simulink model "untitled"  (R2014b)
settings: Solver=ode45  StartTime=0.0  StopTime=0.01  MaxStep=1e-6  RelTol=1e-3
undefined symbols (not defined in the file or in its folder): powergui
libraries: powerlib x15
settings Model: Creator=JPSOLIV  LastModifiedBy=JPSOLIV

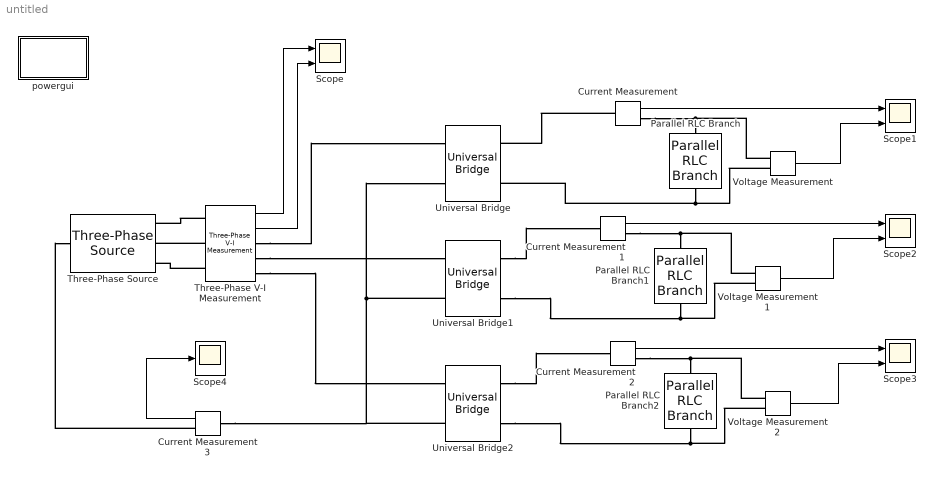
== system untitled ==
  Current Measurement{,1..3} (4 alike) : powerlib/Measurements/Current Measurement  PhasorSimulation=off  OutputType=Complex  PSBequivalent=0
  Parallel RLC Branch : powerlib/Elements/Parallel RLC Branch  LConnTagsString=a  RConnTagsString=__new0  BranchType=RC  Resistance=20  Inductance=1e-3  SetiL0=off  InitialCurrent=0  Capacitance=30e-6  Setx0=off  InitialVoltage=0  Measurements=None
  Parallel RLC Branch1 : powerlib/Elements/Parallel RLC Branch  LConnTagsString=a  RConnTagsString=__new0  BranchType=RC  Resistance=20  Inductance=1e-3  SetiL0=off  InitialCurrent=0  Capacitance=30e-6  Setx0=off  InitialVoltage=0  Measurements=None
  Parallel RLC Branch2 : powerlib/Elements/Parallel RLC Branch  LConnTagsString=a  RConnTagsString=__new0  BranchType=RC  Resistance=20  Inductance=1e-3  SetiL0=off  InitialCurrent=0  Capacitance=30e-6  Setx0=off  InitialVoltage=0  Measurements=None
  Scope{,1..3} (4 alike) : Scope  NumInputPorts=2
      Scope settings: YMin=-600~-200  YMax=400~200
      Scope1 settings: YMin=-0.00169333~0  YMax=20~200
      Scope2 settings: YMin=-5~-5  YMax=5~5  SaveName=ScopeData2
      Scope3 settings: YMin=-5~-5  YMax=5~5  SaveName=ScopeData3
  Scope4 : Scope
      settings: YMin=-10  YMax=15  SaveName=ScopeData4
  Three-Phase V-I Measurement : powerlib/Measurements/Three-Phase V-I Measurement  VoltageMeasurement=phase-to-phase  SetLabelV=off  LabelV=Vabc  Vpu=off  VpuLL=off  CurrentMeasurement=yes  SetLabelI=off  LabelI=Iabc  Ipu=off  Pbase=100e6  Vbase=500e3  OutputType=Complex  PhasorSimulation=off  PSBequivalent=0
  Three-Phase Source : powerlib/Electrical Sources/Three-Phase Source  Voltage=115*sqrt(3)  PhaseAngle=0  Frequency=400  InternalConnection=Yn  SpecifyImpedance=off  Resistance=0.8929e-9  Inductance=16.58e-12  ShortCircuitLevel=100e6  BaseVoltage=115*sqrt(3)  XRratio=7  BusType=swing  Pref=0  Qref=0  Qmin=-inf  Qmax=inf
  Universal Bridge : powerlib/Power Electronics/Universal Bridge  Arms=2  SnubberResistance=1e5  SnubberCapacitance=inf  Device=Diodes  Ron=1e-3  Lon=0  ForwardVoltages="[  0  0  ]"  ForwardVoltage=0  GTOparameters=[ 10e-6 , 20e-6 ]  IGBTparameters=[ 1e-6 , 2e-6 ]  Measurements=None  Measurements_2=None  converterType=Rectifier
  Universal Bridge1 : powerlib/Power Electronics/Universal Bridge  Arms=2  SnubberResistance=1e5  SnubberCapacitance=inf  Device=Diodes  Ron=1e-3  Lon=0  ForwardVoltages="[  0  0  ]"  ForwardVoltage=0  GTOparameters=[ 10e-6 , 20e-6 ]  IGBTparameters=[ 1e-6 , 2e-6 ]  Measurements=None  Measurements_2=None  converterType=Rectifier
  Universal Bridge2 : powerlib/Power Electronics/Universal Bridge  Arms=2  SnubberResistance=1e5  SnubberCapacitance=inf  Device=Diodes  Ron=1e-3  Lon=0  ForwardVoltages="[  0  0  ]"  ForwardVoltage=0  GTOparameters=[ 10e-6 , 20e-6 ]  IGBTparameters=[ 1e-6 , 2e-6 ]  Measurements=None  Measurements_2=None  converterType=Rectifier
  Voltage Measurement : powerlib/Measurements/Voltage Measurement  PhasorSimulation=off  OutputType=Complex  PSBequivalent=0
  Voltage Measurement1 : powerlib/Measurements/Voltage Measurement  PhasorSimulation=off  OutputType=Complex  PSBequivalent=0
  Voltage Measurement2 : powerlib/Measurements/Voltage Measurement  PhasorSimulation=off  OutputType=Complex  PSBequivalent=0
  powergui : Subsystem  Priority=1  AncestorBlock=powerlib/powergui  InitFcn=powergui( 'InitFcn_Callback' , gcb , 0 , [ ] );  StopFcn=powergui( 'StopFcn_Callback' , gcb , 0 , [ ] );  mask(PSB option menu block){SimulationMode=Discrete, SolverType=Tustin/Backward Euler (TBE), SampleTime=5e-8, frequency=60, SPID=off, DisableSnubberDevices=off, DisableRonSwitches=off, DisableVfSwitches=off, SwTol=0, DisplayEquations=off, Interpol=off, methode=off, Ts=100, frequencyindice=0, Pbase=100e6, ErrMax=1e-4, Iterations=50, UnitsV=kV, UnitsW=MW, FunctionMessages=off, echomessages=off, HookPort=off, EnableUseOfTLC=off, x0status=blocks, RestoreLinks=warning, ResistiveCurrentMeasurement=off, Frange=[0:2:500], Ylog=off, Xlog=on, ShowGrid=off, save=off, variable=ZData, structure=0, ZoomFFT=off, StartTime=0.0, cycles=1, DisplayStyle=1, fundamental=60, FreqAxis=off, MaxFrequency=1000, frequencyindicesteady=1, RmsSteady=1, display=off}
      mask prompts: SimulationMode "Simulation type:"; SolverType "Solver type:"; SampleTime "Sample time (s):"; frequency "Phasor frequency (Hz):"; SPID "Enable use of ideal switching devices"; DisableSnubberDevices "Disable snubbers in switching devices"; DisableRonSwitches "Disable On resistance in switching devices (Ron=0)"; DisableVfSwitches "Disable Forward voltage in switching devices (Vf=0)"; SwTol "Switch tolerance"; DisplayEquations "Display circuit differential equations"; Interpol "Interpolate"; methode "Store state-space matrices"; Ts "Buffer size (MBytes)"; frequencyindice "Load flow frequency (Hz):"; Pbase "Base power Pbase (VA):"; ErrMax "PQ tolerance (pu):"; Iterations "Max iterations:"; UnitsV "Voltage units"; UnitsW "Power units"; FunctionMessages "Disable SimPowerSystems warnings"; echomessages "Display SimPowerSystems compilation messages"; HookPort "Add a hook port to the powergui block"; EnableUseOfTLC "Use TLC file when in Accelerator Simulation Mode and for code generation"; x0status "Start simulation with initial electrical states from:"; RestoreLinks "Restore disabled links of SimPowerSystems blocks:"; ResistiveCurrentMeasurement "Use non ideal current measurement blocks (1e-4Ohm internal resistance)"; Frange "Frequency Range"; Ylog "Log impedance"; Xlog "log Frequency"; ShowGrid "grid"; save "Save Data To Workspace"; variable "Variable Name"; structure "Structure Name (PSBFFTSCOPE)"; ZoomFFT "ZoomFFT (PSBFFTSCOPE)"; StartTime "Start Time (PSBFFTSCOPE)"; cycles "Cycles (PSBFFTSCOPE)"; DisplayStyle "Display style (PSBFFTSCOPE)"; fundamental "Fundamental (PSBFFTSCOPE)"; FreqAxis "Frequency Axis (PSBFFTSCOPE)"; MaxFrequency "Max Frequency (PSBFFTSCOPE)"; frequencyindicesteady "Frequency indice (STEADYSTATE)"; RmsSteady "RMS display (STEADYSTATE)"; display "Display Results"
      mask help: Set simulation type, simulation parameters, and preferences
      mask init:
      | message = powergui('MaskInitialization',gcb,SimulationMode,SampleTime);
      settings: CopyFcn=powergui( 'Copy_Callback' , gcb , 0 , [ ] );  ModelCloseFcn=powergui( 'CloseButton_Callback' , gcb , [ ] , [ ] );  NameChangeFcn=powergui( 'NameChangeFcn_Callback' , gcb , 0 , [ ] );  OpenFcn=powergui(gcb,'Open')
      settings: DeleteFcn=|
      | % see geck 675031 powergui( 'Copy_Callback' , gcb , 1 , [ ] );
      | 
      | powergui( 'CloseButton_Callback' , gcb , [ ] , [ ] );
      settings: PreSaveFcn=|
      | powergui( 'PreSaveFcn_Callback' , gcb , [ ] , [ ] );
      | powergui( 'CloseButton_Callback' , gcb , [ ] , [ ] );
      mask Help: helpview(psbhelp)
      mask TypeOptions SimulationMode: Continuous | Discrete | Phasor
      mask Callback SimulationMode: powergui('SimulationType',[],[],gcb);
      mask TypeOptions SolverType: Tustin/Backward Euler (TBE) | Tustin | Backward Euler
      mask Callback SolverType: powergui('SolverType',[],[],gcb);
      mask Callback SPID: powergui('SPID',[],[],gcb);
      mask Callback Interpol: powergui('INTERPOLATE',[],[],gcb);
      mask Callback methode: powergui('STORE',[],[],gcb);
      mask TypeOptions UnitsV: V | kV
      mask TypeOptions UnitsW: W | kW | MW
      mask Callback HookPort: powergui('HookPort',[],[],gcb);
      mask TypeOptions x0status: blocks | steady | zero
      mask TypeOptions RestoreLinks: yes | warning | no
      mask DialogControl Advanced Prompt: Advanced settings (Tustin solver)
      mask Display: color('blue'),disp(message)
  wires:
  Three-Phase V-I Measurement/1 -> Scope/1
  Three-Phase V-I Measurement/2 -> Scope/2
  Current Measurement/1 -> Scope1/1
  Voltage Measurement/1 -> Scope1/2
  Current Measurement1/1 -> Scope2/1
  Voltage Measurement1/1 -> Scope2/2
  Current Measurement2/1 -> Scope3/1
  Voltage Measurement2/1 -> Scope3/2
  Current Measurement3/1 -> Scope4/1
  connections:
  Universal Bridge1/LConn2 -- Current Measurement3/LConn1 -- Universal Bridge2/LConn2 -- Universal Bridge/LConn2
  Parallel RLC Branch/RConn1 -- Universal Bridge/RConn2 -- Voltage Measurement/LConn2
  Three-Phase V-I Measurement/LConn1 -- Three-Phase Source/RConn1
  Three-Phase V-I Measurement/LConn2 -- Three-Phase Source/RConn2
  Three-Phase V-I Measurement/LConn3 -- Three-Phase Source/RConn3
  Three-Phase V-I Measurement/RConn1 -- Universal Bridge/LConn1
  Three-Phase V-I Measurement/RConn2 -- Universal Bridge1/LConn1
  Three-Phase V-I Measurement/RConn3 -- Universal Bridge2/LConn1
  Current Measurement/RConn1 -- Voltage Measurement/LConn1 -- Parallel RLC Branch/LConn1
  Current Measurement/LConn1 -- Universal Bridge/RConn1
  Parallel RLC Branch1/RConn1 -- Universal Bridge1/RConn2 -- Voltage Measurement1/LConn2
  Parallel RLC Branch1/LConn1 -- Current Measurement1/RConn1 -- Voltage Measurement1/LConn1
  Universal Bridge1/RConn1 -- Current Measurement1/LConn1
  Parallel RLC Branch2/RConn1 -- Universal Bridge2/RConn2 -- Voltage Measurement2/LConn2
  Parallel RLC Branch2/LConn1 -- Current Measurement2/RConn1 -- Voltage Measurement2/LConn1
  Universal Bridge2/RConn1 -- Current Measurement2/LConn1
  Current Measurement3/RConn1 -- Three-Phase Source/LConn1

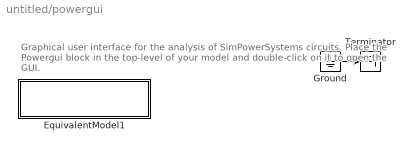
== system untitled/powergui ==
  note: Graphical user interface for the analysis of  SimPowerSystems circuits.
      | Place the Powergui block in the top-level of your model and double-click
      | on it to open the GUI.
  EquivalentModel1 : Subsystem
      mask init:
      | S  = GetDataForEquivalentModel('Discrete',gcbh);
      mask Display:
      | color('red')
      | disp('EQUIVALENT CIRCUIT\nDiscrete')
  Ground : Ground
  Terminator : Terminator
  wires:
  Ground/1 -> Terminator/1

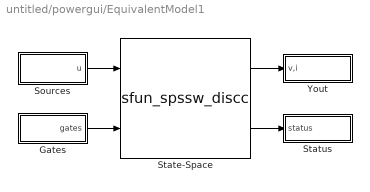
== system untitled/powergui/EquivalentModel1 ==
  Gates : Subsystem
  Sources : Subsystem
  State-Space : S-Function  FunctionName=sfun_spssw_discc  Parameters=S.Ts,S.A, S.B, S.C, S.D, S.x0, S.EnableUseOfTLC,S.SwitchResistance ,S.SwitchType, S.SwitchGateInitialValue, S.OutputsToResetToZero, S.TBEON  EnableBusSupport=off
  Status : Subsystem
  Yout : Subsystem
  wires:
  State-Space/1 -> Yout/1(v,i)
  State-Space/2 -> Status/1(status)
  Sources/1(u) -> State-Space/1
  Gates/1(gates) -> State-Space/2

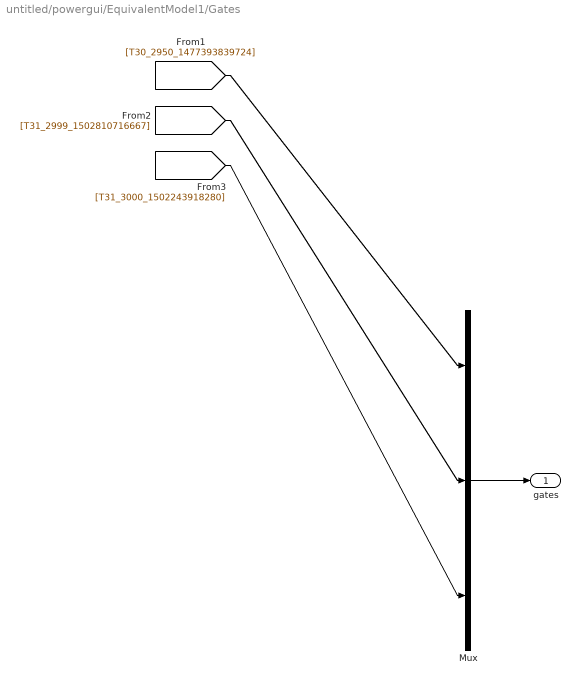
== system untitled/powergui/EquivalentModel1/Gates ==
  Mux : Mux  Inputs=[4 4 4]
  gates : Outport
  wires:
  Mux/1 -> gates/1
  [T30_2950_1477393839724] -> Mux/1
  [T31_2999_1502810716667] -> Mux/2
  [T31_3000_1502243918280] -> Mux/3

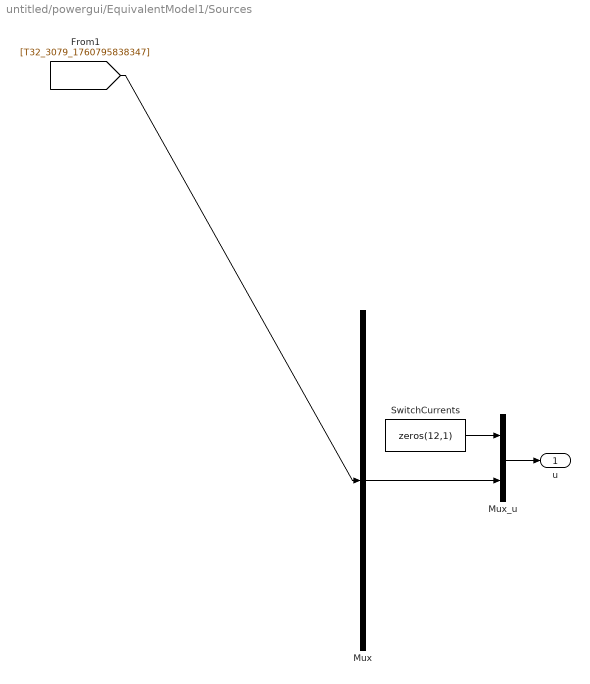
== system untitled/powergui/EquivalentModel1/Sources ==
  Mux : Mux  Inputs=1
  Mux_u : Mux  Inputs=[12 3]
  SwitchCurrents : Constant  Value=zeros(12,1)
  u : Outport
  wires:
  Mux/1 -> Mux_u/2
  SwitchCurrents/1 -> Mux_u/1
  Mux_u/1 -> u/1
  [T32_3079_1760795838347] -> Mux/1

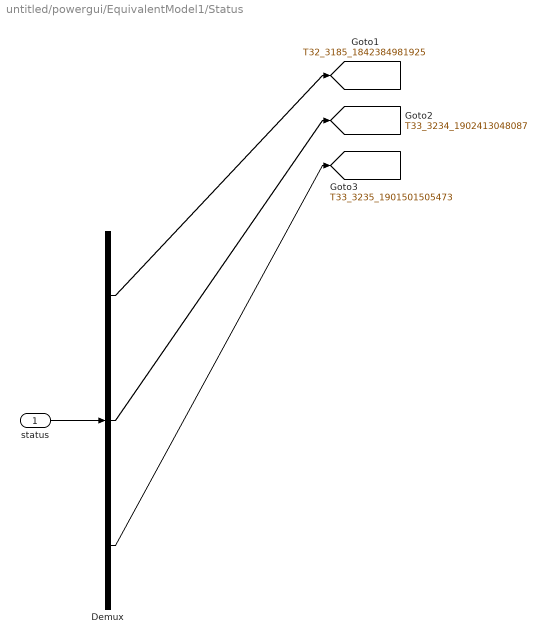
== system untitled/powergui/EquivalentModel1/Status ==
  status : Inport
  Demux : Demux  Outputs=[4 4 4]
  tag scope: T32_3185_1842384981925=global, T33_3234_1902413048087=global, T33_3235_1901501505473=global
  wires:
  status/1 -> Demux/1
  Demux/1 -> [T32_3185_1842384981925]
  Demux/2 -> [T33_3234_1902413048087]
  Demux/3 -> [T33_3235_1901501505473]

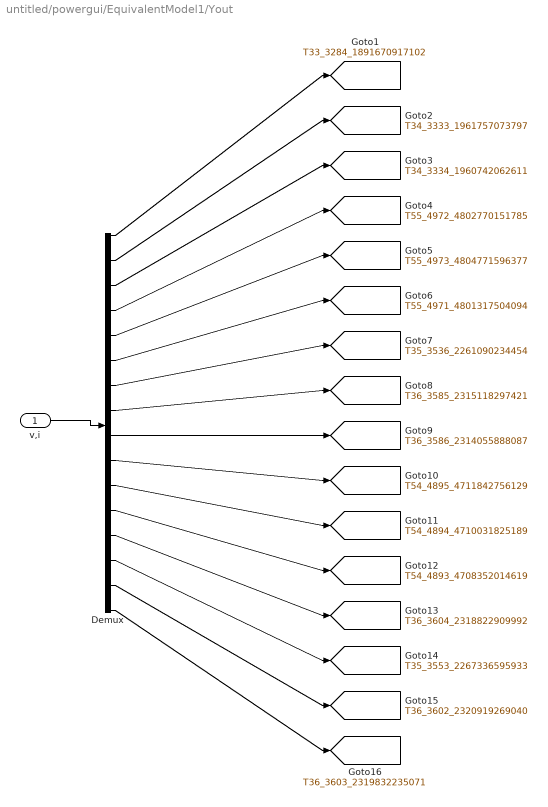
== system untitled/powergui/EquivalentModel1/Yout ==
  v,i : Inport
  Demux : Demux  Outputs=[4 4 4 1 1 1 1 1 1 1 1 1 1 1 1 1]
  tag scope: T33_3284_1891670917102=global, T34_3333_1961757073797=global, T34_3334_1960742062611=global, T35_3536_2261090234454=global, T35_3553_2267336595933=global, T36_3585_2315118297421=global, T36_3586_2314055888087=global, T36_3602_2320919269040=global, T36_3603_2319832235071=global, T36_3604_2318822909992=global, T54_4893_4708352014619=global, T54_4894_4710031825189=global, T54_4895_4711842756129=global, T55_4971_4801317504094=global, T55_4972_4802770151785=global, T55_4973_4804771596377=global
  wires:
  v,i/1 -> Demux/1
  Demux/1 -> [T33_3284_1891670917102]
  Demux/2 -> [T34_3333_1961757073797]
  Demux/3 -> [T34_3334_1960742062611]
  Demux/4 -> [T55_4972_4802770151785]
  Demux/5 -> [T55_4973_4804771596377]
  Demux/6 -> [T55_4971_4801317504094]
  Demux/7 -> [T35_3536_2261090234454]
  Demux/8 -> [T36_3585_2315118297421]
  Demux/9 -> [T36_3586_2314055888087]
  Demux/10 -> [T54_4895_4711842756129]
  Demux/11 -> [T54_4894_4710031825189]
  Demux/12 -> [T54_4893_4708352014619]
  Demux/13 -> [T36_3604_2318822909992]
  Demux/14 -> [T35_3553_2267336595933]
  Demux/15 -> [T36_3602_2320919269040]
  Demux/16 -> [T36_3603_2319832235071]
